simulink library "ControllersLib"  (R2022b)
settings: Solver=VariableStepAuto  StartTime=0.0  StopTime=10.0  RelTol=1e-3
undefined symbols (not defined in the file or in its folder): SimIn
libraries: ComponentsLib x5
settings Model: Creator=tbritton  LastModifiedBy=macheson
settings SolverCC: AlgebraicLoopSolver=TrustRegion
settings DebuggingCC: UnconnectedInputMsg=warning  UnconnectedOutputMsg=warning  UnconnectedLineMsg=warning  SFMachineParentedDataDiag=warning
settings ModelReferenceCC: EnableRefExpFcnMdlSchedulingChecks=on
settings RTWCC: DLArmComputeVersion=19.05

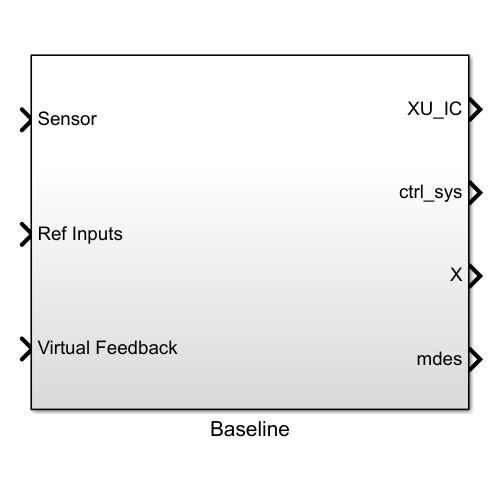
[thumbnail: Simulink's stored preview of the top-level diagram]
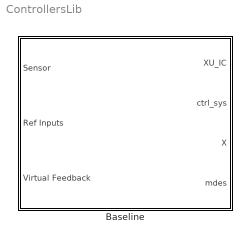
== system ControllersLib ==
  Baseline : Subsystem

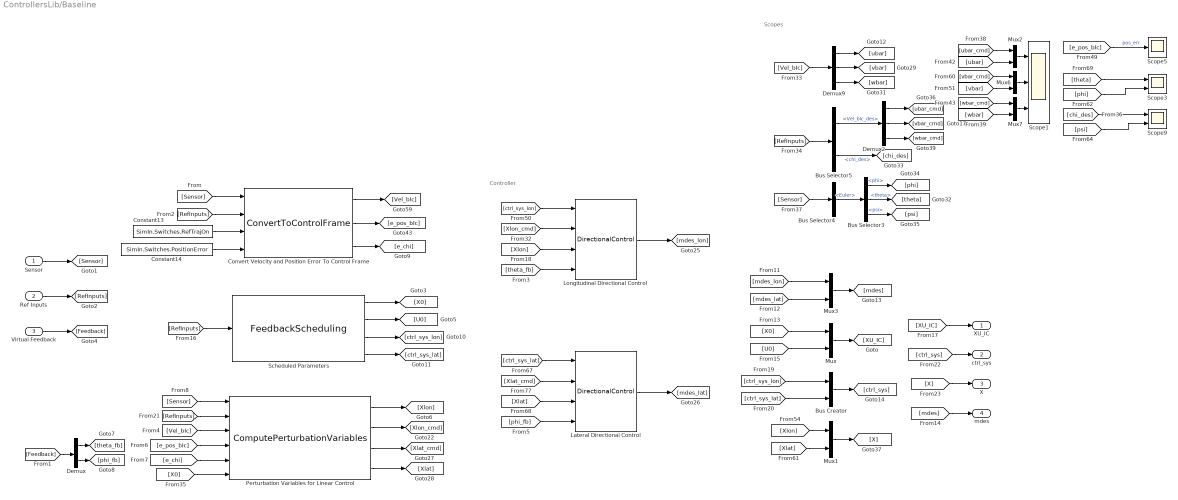
== system ControllersLib/Baseline ==
  note: Controller
  note: Scopes
  Sensor : Inport  OutDataTypeStr=Bus: SensorBus
  Ref Inputs : Inport  Port=2  OutDataTypeStr=Bus: BUS_REF_INPUT
  Virtual Feedback : Inport  Port=3
  Bus Creator : BusCreator  Inputs=2
  Bus Selector3 : BusSelector  OutputSignals=phi,theta,psi
  Bus Selector4 : BusSelector  OutputSignals=Euler
  Bus Selector5 : BusSelector  OutputSignals=Vel_bIc_des,chi_des
  Constant13 : Constant  Value=SimIn.Switches.RefTrajOn
  Constant14 : Constant  Value=SimIn.Switches.PositionError
  Convert Velocity and Position Error To Control Frame : ComponentsLib/ConvertToControlFrame  SystemSampleTime=-1  VariantActivationTime=update diagram  Latency=0  AutoFrameSizeCalculation=off
      settings: SourceProductName=GUAM Controller Blockset
  Demux : Demux  Outputs=2
  Demux2 : Demux  Outputs=3
  Demux9 : Demux  Outputs=3
  Lateral Directional Control : ComponentsLib/DirectionalControl  SystemSampleTime=-1  VariantActivationTime=update diagram  Latency=0  AutoFrameSizeCalculation=off
      settings: SourceProductName=GUAM Controller Blockset
  Longitudinal Directional Control : ComponentsLib/DirectionalControl  SystemSampleTime=-1  VariantActivationTime=update diagram  Latency=0  AutoFrameSizeCalculation=off
      settings: SourceProductName=GUAM Controller Blockset
  Mux{,1..3,6..7} (6 alike) : Mux  Inputs=2
  Perturbation Variables for Linear Control : ComponentsLib/ComputePerturbationVariables  SystemSampleTime=-1  VariantActivationTime=update diagram  Latency=0  AutoFrameSizeCalculation=off
      settings: SourceProductName=GUAM Controller Blockset
  Scheduled Parameters : ComponentsLib/FeedbackScheduling  SystemSampleTime=-1  VariantActivationTime=update diagram  Latency=0  AutoFrameSizeCalculation=off
      settings: SourceProductName=GUAM Controller Blockset
  Scope1 : Scope  NumInputPorts=3
  Scope3 : Scope  NumInputPorts=2
  Scope5 : Scope
  Scope9 : Scope  NumInputPorts=2
  XU_IC : Outport
  ctrl_sys : Outport  Port=2
  X : Outport  Port=3
  mdes : Outport  Port=4
  wires:
  [X0] -> Perturbation Variables for Linear Control/6
  Perturbation Variables for Linear Control/1 -> [Xlon]
  [Sensor] -> Perturbation Variables for Linear Control/1
  Perturbation Variables for Linear Control/3 -> [Xlat_cmd]
  Sensor/1 -> [Sensor]
  Scheduled Parameters/1 -> [X0]
  Ref Inputs/1 -> [RefInputs]
  [RefInputs] -> Convert Velocity and Position Error To Control Frame/2
  Convert Velocity and Position Error To Control Frame/1 -> [Vel_bIc]
  Convert Velocity and Position Error To Control Frame/2 -> [e_pos_bIc]
  Scheduled Parameters/3 -> [ctrl_sys_lon]
  [e_pos_bIc] -> Perturbation Variables for Linear Control/4
  Perturbation Variables for Linear Control/4 -> [Xlat]
  [RefInputs] -> Scheduled Parameters/1
  Perturbation Variables for Linear Control/2 -> [Xlon_cmd]
  Convert Velocity and Position Error To Control Frame/3 -> [e_chi]
  [Sensor] -> Convert Velocity and Position Error To Control Frame/1
  [Vel_bIc] -> Perturbation Variables for Linear Control/3
  Constant13/1 -> Convert Velocity and Position Error To Control Frame/3
  [RefInputs] -> Perturbation Variables for Linear Control/2
  Constant14/1 -> Convert Velocity and Position Error To Control Frame/4
  [e_chi] -> Perturbation Variables for Linear Control/5
  Scheduled Parameters/2 -> [U0]
  Scheduled Parameters/4 -> [ctrl_sys_lat]
  [Xlon_cmd] -> Longitudinal Directional Control/2
  Lateral Directional Control/1 -> [mdes_lat]
  [ctrl_sys_lat] -> Lateral Directional Control/1
  [ctrl_sys_lon] -> Longitudinal Directional Control/1
  Longitudinal Directional Control/1 -> [mdes_lon]
  [Xlat] -> Lateral Directional Control/3
  [Xlon] -> Longitudinal Directional Control/3
  [Xlat_cmd] -> Lateral Directional Control/2
  Virtual Feedback/1 -> [Feedback]
  [Feedback] -> Demux/1
  Demux/2 -> [phi_fb]
  Demux/1 -> [theta_fb]
  [theta_fb] -> Longitudinal Directional Control/4
  [phi_fb] -> Lateral Directional Control/4
  [mdes_lon] -> Mux3/1
  [mdes_lat] -> Mux3/2
  Mux3/1 -> [mdes]
  [mdes] -> mdes/1
  [X0] -> Mux/1
  [U0] -> Mux/2
  Mux/1 -> [XU_IC]
  [XU_IC] -> XU_IC/1
  [ctrl_sys_lon] -> Bus Creator/1
  [ctrl_sys_lat] -> Bus Creator/2
  Bus Creator/1 -> [ctrl_sys]
  [ctrl_sys] -> ctrl_sys/1
  Mux1/1 -> [X]
  [Xlon] -> Mux1/1
  [Xlat] -> Mux1/2
  [X] -> X/1
  [ubar] -> Mux2/2
  Bus Selector4/1 -> Bus Selector3/1  "<Euler>"
  Bus Selector5/2 -> [chi_des]  "<chi_des>"
  Demux2/3 -> [wbar_cmd]
  Demux2/2 -> [vbar_cmd]
  [wbar_cmd] -> Mux7/1
  Bus Selector3/2 -> [theta]  "<theta>"
  Demux9/3 -> [wbar]
  Bus Selector5/1 -> Demux2/1  "<Vel_bIc_des>"
  [Sensor] -> Bus Selector4/1
  Mux2/1 -> Scope1/1
  [wbar] -> Mux7/2
  Mux6/1 -> Scope1/2
  Mux7/1 -> Scope1/3
  [chi_des] -> Scope9/1
  [vbar_cmd] -> Mux6/1
  [e_pos_bIc] -> Scope5/1  "pos_err"
  [theta] -> Scope3/1
  Demux9/2 -> [vbar]
  Demux9/1 -> [ubar]
  [psi] -> Scope9/2
  [RefInputs] -> Bus Selector5/1
  Demux2/1 -> [ubar_cmd]
  Bus Selector3/1 -> [phi]  "<phi>"
  Bus Selector3/3 -> [psi]  "<psi>"
  [ubar_cmd] -> Mux2/1
  [vbar] -> Mux6/2
  [phi] -> Scope3/2
  [Vel_bIc] -> Demux9/1
